simulink model "control_para"  (R2016b)
settings: Solver=VariableStepAuto  StartTime=0.0  StopTime=10.0  RelTol=1e-3
settings Model: Creator=limu  LastModifiedBy=limu

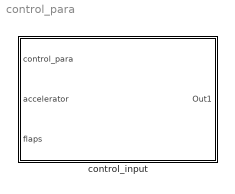
== system control_para ==
  control_input : Subsystem

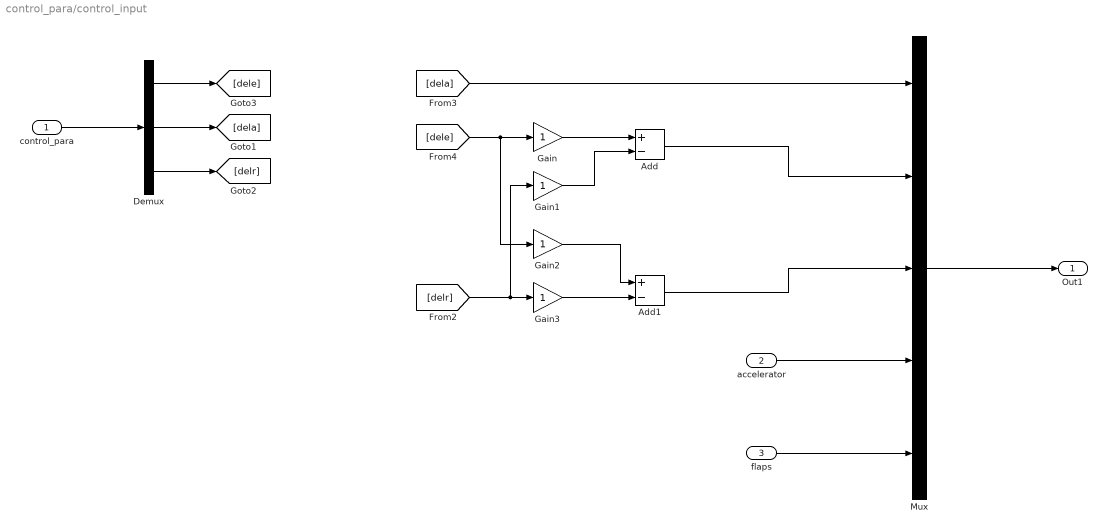
== system control_para/control_input ==
  control_para : Inport
  accelerator : Inport  Port=2
  flaps : Inport  Port=3
  Add : Sum  Inputs=+-
  Add1 : Sum  Inputs=+-
  Demux : Demux  Outputs=3
  Gain{,1..3} (4 alike) : Gain
  Mux : Mux  Inputs=5
  Out1 : Outport
  wires:
  control_para/1 -> Demux/1
  Demux/1 -> [dele]
  Demux/2 -> [dela]
  Demux/3 -> [delr]
  Mux/1 -> Out1/1
  [dela] -> Mux/1
  [dele] -> Gain2/1, Gain/1
  [delr] -> Gain1/1, Gain3/1
  Gain/1 -> Add/1
  Gain1/1 -> Add/2
  Gain2/1 -> Add1/1
  Gain3/1 -> Add1/2
  Add1/1 -> Mux/3
  Add/1 -> Mux/2
  accelerator/1 -> Mux/4
  flaps/1 -> Mux/5
